simulink model "rate_limit_prove"  (R2014b)
settings: Solver=FixedStepDiscrete  StartTime=0.0  StopTime=10.0  FixedStep=0.01  RelTol=1e-3
undefined symbols (not defined in the file): sldvsubsys
libraries: sldvlib x12, simulink x6
settings Model: ModifiedByFormat=Natasha  Creator=Natasha  LastModifiedBy=Natasha
settings DebuggingCC: UnderspecifiedInitializationDetection=Classic  MergeDetectMultiDrivingBlocksExec=none
settings ConfigComp: Description=Design Verifier Custom Configuration Component  DVMode=PropertyProving  DVMaxProcessTime=1200  DVMaxTestCaseSteps=500  DVTestSuiteOptimization=CombinedObjectives (Nonlinear Extended)  DVDetectActiveLogic=on

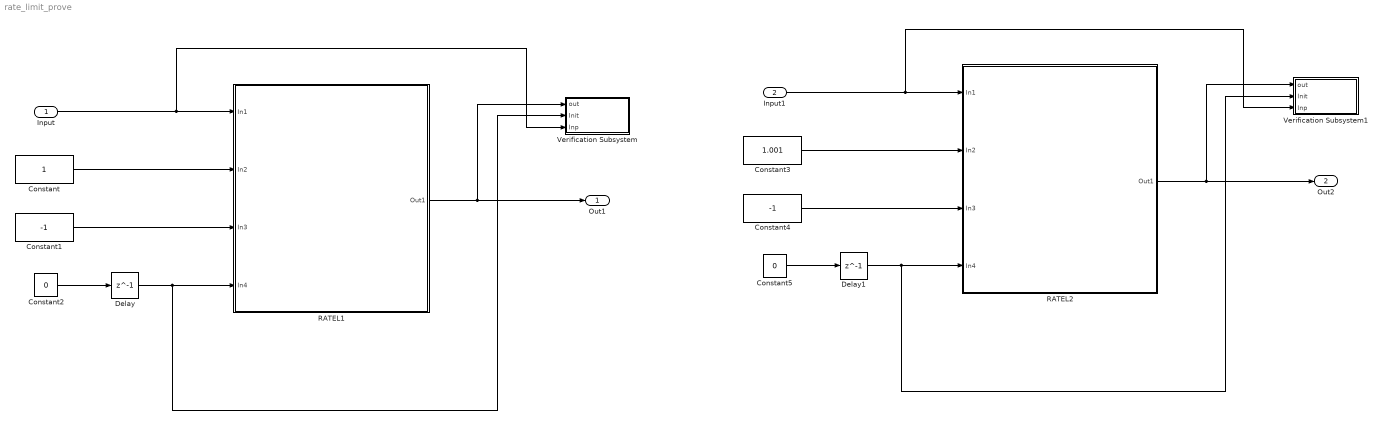
== system rate_limit_prove ==
  Input : Inport
  Input1 : Inport  Port=2
  Constant : Constant  OutDataTypeStr=single
  Constant1 : Constant  Value=-1  OutDataTypeStr=single
  Constant2 : Constant  Value=0  OutDataTypeStr=boolean
  Constant3 : Constant  Value=1.001  OutDataTypeStr=single
  Constant4 : Constant  Value=-1  OutDataTypeStr=single
  Constant5 : Constant  Value=0  OutDataTypeStr=boolean
  Delay : Delay  DelayLength=1  InitialCondition=1
  Delay1 : Delay  DelayLength=1  InitialCondition=1
  RATEL1 : Subsystem  Description=Rate Limiter  mask{DT=0.01}
      mask prompts: DT "Input the Sample Time"
      settings: AttributesFormatString=%<Description>\nSample Time = %<DT>
      mask Display:
      | port_label('output', 1, 'Rate limited')
      | port_label('input', 1, 'Input')
      | port_label('input', 2, 'Rising Limit')
      | port_label('input', 3, 'Falling Limit')
      | port_label('input', 4, 'Init')
      | patch([0.35 .5 0.65], [0 .3 0], [0 1 0])
      | text(0.4,0.1, 'Safe')
  RATEL2 : Subsystem  Description=Rate Limiter  mask{DT=0.01}
      mask prompts: DT "Input the Sample Time"
      settings: AttributesFormatString=%<Description>\nSample Time = %<DT>
      mask Display:
      | port_label('output', 1, 'Rate limited')
      | port_label('input', 1, 'Input')
      | port_label('input', 2, 'Rising Limit')
      | port_label('input', 3, 'Falling Limit')
      | port_label('input', 4, 'Init')
      | patch([0.35 .5 0.65], [0 .3 0], [0 1 0])
      | text(0.4,0.1, 'Safe')
  Verification Subsystem : Subsystem  Tag=VerificationSubsystem  DisableCoverage=on  LoadFcn=sldvsubsys('check')  TreatAsAtomicUnit=on  SimViewingDevice=on  mask(VerificationSubsystem){}
      mask init:
      | sldvsubsys('maskInit');
      settings: CopyFcn=sldvsubsys('copy');  OpenFcn=open_system(gcb,'force');
      settings: PreSaveFcn=|
      | set_param(gcb,'SimViewingDevice','on');
      | sldvsubsys('check');
      mask Help: helpview(fullfile(docroot,'toolbox','sldv','sldv.map'),'verificationsubsystem')
      mask Display: image(imread('sldvicon_versubsys.png','BackGroundColor',[1 1 1]),'center');
  Verification Subsystem1 : Subsystem  Tag=VerificationSubsystem  DisableCoverage=on  LoadFcn=sldvsubsys('check')  TreatAsAtomicUnit=on  SimViewingDevice=on  mask(VerificationSubsystem){}
      mask init:
      | sldvsubsys('maskInit');
      settings: CopyFcn=sldvsubsys('copy');  OpenFcn=open_system(gcb,'force');
      settings: PreSaveFcn=|
      | set_param(gcb,'SimViewingDevice','on');
      | sldvsubsys('check');
      mask Help: helpview(fullfile(docroot,'toolbox','sldv','sldv.map'),'verificationsubsystem')
      mask Display: image(imread('sldvicon_versubsys.png','BackGroundColor',[1 1 1]),'center');
  Out1 : Outport
  Out2 : Outport  Port=2
  wires:
  Constant/1 -> RATEL1/2(In2)
  Constant1/1 -> RATEL1/3(In3)
  Constant2/1 -> Delay/1
  RATEL1/1(Out1) -> Verification Subsystem/1(out), Out1/1
  Delay/1 -> Verification Subsystem/2(Init), RATEL1/4(In4)
  Input/1 -> RATEL1/1(In1), Verification Subsystem/3(Inp)
  Constant3/1 -> RATEL2/2(In2)
  Constant4/1 -> RATEL2/3(In3)
  Constant5/1 -> Delay1/1
  RATEL2/1(Out1) -> Verification Subsystem1/1(out), Out2/1
  Delay1/1 -> Verification Subsystem1/2(Init), RATEL2/4(In4)
  Input1/1 -> Verification Subsystem1/3(Inp), RATEL2/1(In1)

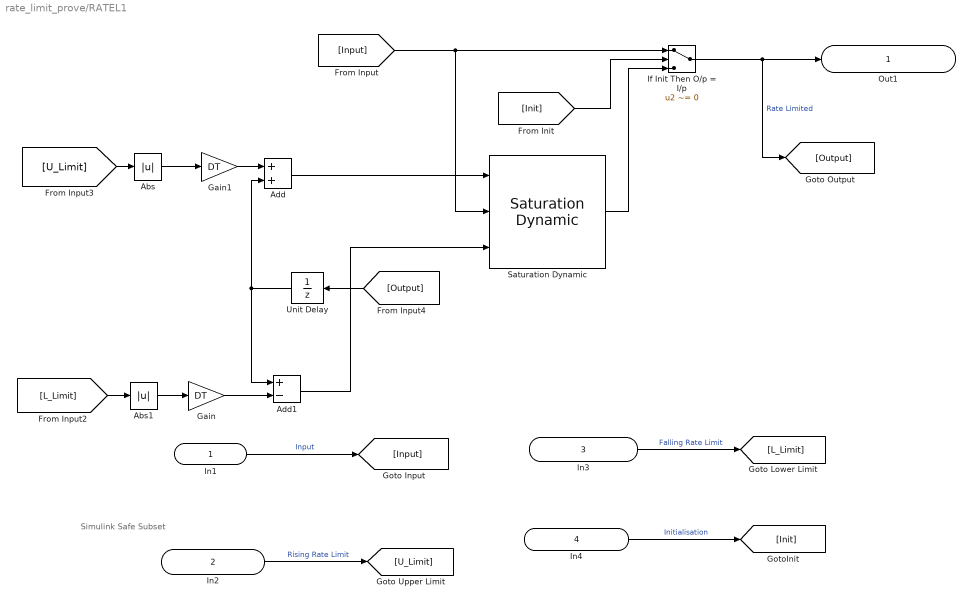
== system rate_limit_prove/RATEL1 ==
  note: Simulink
      | Safe
      | Subset
  In1 : Inport  Description=Input Signal  OutDataTypeStr=single
      settings: AttributesFormatString=%<Description>\nPort No = %<Port>\nSample Time = %<SampleTime>\nSignal Type = %<SignalType>
  In2 : Inport  Description=Rising Limit  Port=2  OutDataTypeStr=single
      settings: AttributesFormatString=%<Description>\nPort No = %<Port>\nSample Time = %<SampleTime>\nSignal Type = %<SignalType>
  In3 : Inport  Description=Falling Limit  Port=3  OutDataTypeStr=single
      settings: AttributesFormatString=%<Description>\nPort No = %<Port>\nSample Time = %<SampleTime>\nSignal Type = %<SignalType>
  In4 : Inport  Description=Initialise  Port=4  OutDataTypeStr=boolean
      settings: AttributesFormatString=%<Description>\nPort No = %<Port>\nSample Time = %<SampleTime>\nSignal Type = %<SignalType>
  Abs : Abs
      settings: AttributesFormatString=ST = %<SampleTime>
  Abs1 : Abs
      settings: AttributesFormatString=ST = %<SampleTime>
  Add : Sum
      settings: AttributesFormatString=ST = %<SampleTime>
  Add1 : Sum  Inputs=+-
      settings: AttributesFormatString=ST = %<SampleTime>
  Gain : Gain  Gain=DT
  Gain1 : Gain  Gain=DT
  If Init Then O/p = I/p : Switch  Criteria=u2 ~= 0  Threshold=0.5  ZeroCross=off
      settings: AttributesFormatString=ST = %<SampleTime>\nThreshold = %<Threshold>\n%<Criteria>
  Saturation Dynamic : simulink/Discontinuities/Saturation Dynamic  OutMin=[]  OutMax=[]  OutDataTypeStr=Inherit: Same as second input  OutDataType=fixdt(1, 16)  OutScaling=2^-10  DoSatur=off
  Unit Delay : UnitDelay  SampleTime=-1
      settings: AttributesFormatString=ST = %<SampleTime>\nInitial = %<X0>
  Out1 : Outport  Description=Output Signal
      settings: AttributesFormatString=%<Description>\nPort No = %<Port>\nSample Time = %<SampleTime>\nSignal Type = %<SignalType>
  wires:
  Add1/1 -> Saturation Dynamic/3
  Add/1 -> Saturation Dynamic/1
  [Output] -> Unit Delay/1
  Gain1/1 -> Add/1
  [U_Limit] -> Abs/1
  Unit Delay/1 -> Add1/1, Add/2
  Gain/1 -> Add1/2
  [L_Limit] -> Abs1/1
  Saturation Dynamic/1 -> If Init Then O/p = I/p/3
  If Init Then O/p = I/p/1 -> [Output], Out1/1  "Rate Limited"
  [Init] -> If Init Then O/p = I/p/2
  In4/1 -> [Init]  "Initialisation"
  In3/1 -> [L_Limit]  "Falling Rate Limit"
  In2/1 -> [U_Limit]  "Rising Rate Limit"
  In1/1 -> [Input]  "Input"
  Abs/1 -> Gain1/1
  Abs1/1 -> Gain/1
  [Input] -> If Init Then O/p = I/p/1, Saturation Dynamic/2

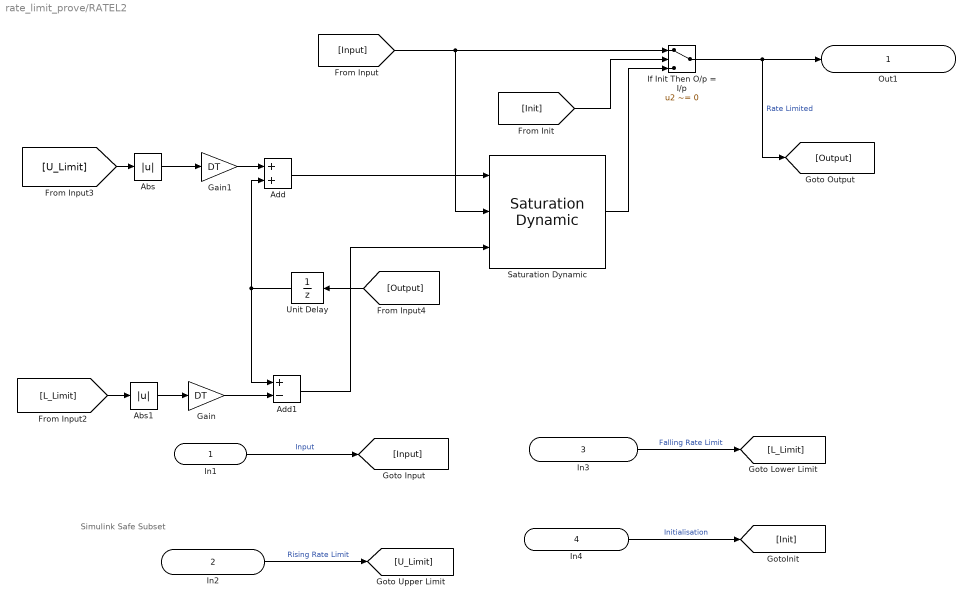
== system rate_limit_prove/RATEL2 ==
  note: Simulink
      | Safe
      | Subset
  In1 : Inport  Description=Input Signal  OutDataTypeStr=single
      settings: AttributesFormatString=%<Description>\nPort No = %<Port>\nSample Time = %<SampleTime>\nSignal Type = %<SignalType>
  In2 : Inport  Description=Rising Limit  Port=2  OutDataTypeStr=single
      settings: AttributesFormatString=%<Description>\nPort No = %<Port>\nSample Time = %<SampleTime>\nSignal Type = %<SignalType>
  In3 : Inport  Description=Falling Limit  Port=3  OutDataTypeStr=single
      settings: AttributesFormatString=%<Description>\nPort No = %<Port>\nSample Time = %<SampleTime>\nSignal Type = %<SignalType>
  In4 : Inport  Description=Initialise  Port=4  OutDataTypeStr=boolean
      settings: AttributesFormatString=%<Description>\nPort No = %<Port>\nSample Time = %<SampleTime>\nSignal Type = %<SignalType>
  Abs : Abs
      settings: AttributesFormatString=ST = %<SampleTime>
  Abs1 : Abs
      settings: AttributesFormatString=ST = %<SampleTime>
  Add : Sum
      settings: AttributesFormatString=ST = %<SampleTime>
  Add1 : Sum  Inputs=+-
      settings: AttributesFormatString=ST = %<SampleTime>
  Gain : Gain  Gain=DT
  Gain1 : Gain  Gain=DT
  If Init Then O/p = I/p : Switch  Criteria=u2 ~= 0  Threshold=0.5  ZeroCross=off
      settings: AttributesFormatString=ST = %<SampleTime>\nThreshold = %<Threshold>\n%<Criteria>
  Saturation Dynamic : simulink/Discontinuities/Saturation Dynamic  OutMin=[]  OutMax=[]  OutDataTypeStr=Inherit: Same as second input  OutDataType=fixdt(1, 16)  OutScaling=2^-10  DoSatur=off
  Unit Delay : UnitDelay  SampleTime=-1
      settings: AttributesFormatString=ST = %<SampleTime>\nInitial = %<X0>
  Out1 : Outport  Description=Output Signal
      settings: AttributesFormatString=%<Description>\nPort No = %<Port>\nSample Time = %<SampleTime>\nSignal Type = %<SignalType>
  wires:
  Add1/1 -> Saturation Dynamic/3
  Add/1 -> Saturation Dynamic/1
  [Output] -> Unit Delay/1
  Gain1/1 -> Add/1
  [U_Limit] -> Abs/1
  Unit Delay/1 -> Add1/1, Add/2
  Gain/1 -> Add1/2
  [L_Limit] -> Abs1/1
  Saturation Dynamic/1 -> If Init Then O/p = I/p/3
  If Init Then O/p = I/p/1 -> [Output], Out1/1  "Rate Limited"
  [Init] -> If Init Then O/p = I/p/2
  In4/1 -> [Init]  "Initialisation"
  In3/1 -> [L_Limit]  "Falling Rate Limit"
  In2/1 -> [U_Limit]  "Rising Rate Limit"
  In1/1 -> [Input]  "Input"
  Abs/1 -> Gain1/1
  Abs1/1 -> Gain/1
  [Input] -> If Init Then O/p = I/p/1, Saturation Dynamic/2

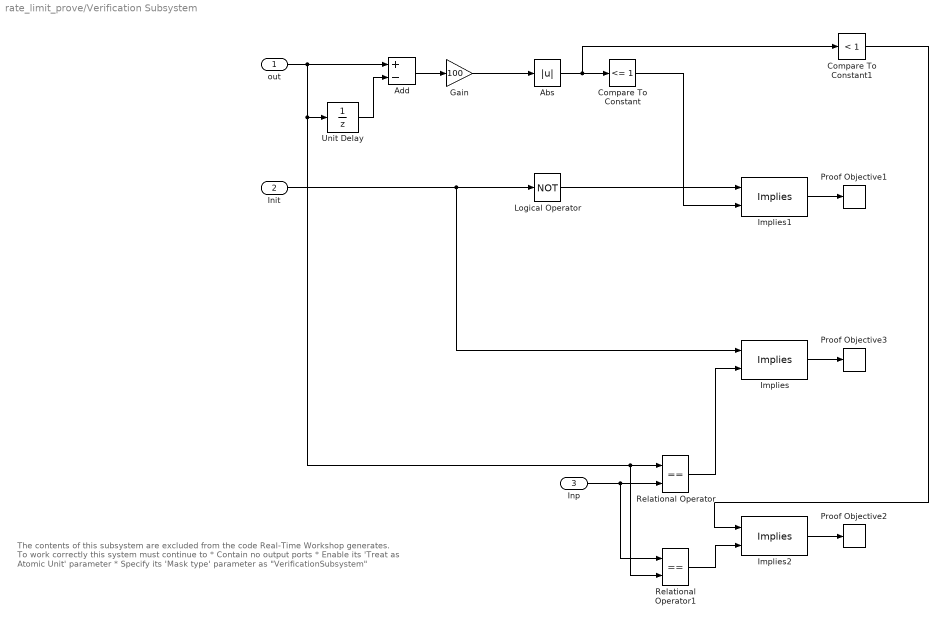
== system rate_limit_prove/Verification Subsystem ==
  note: The contents of this subsystem are excluded from the code Real-Time
      | Workshop generates.
      |
      | To work correctly this system must continue to
      | * Contain no output ports
      | * Enable its 'Treat as Atomic Unit' parameter
      | * Specify its 'Mask type' parameter as "VerificationSubsystem"
  out : Inport
  Init : Inport  Port=2
  Inp : Inport  Port=3
  Abs : Abs
  Add : Sum  Inputs=+-
  Compare To Constant : simulink/Logic and Bit Operations/Compare To Constant  relop=<=  const=1  OutDataTypeStr=boolean
  Compare To Constant1 : simulink/Logic and Bit Operations/Compare To Constant  relop=<  const=1  OutDataTypeStr=boolean
  Gain : Gain  Gain=100
  Implies : sldvlib/Verification Utilities/Implies
  Implies1 : sldvlib/Verification Utilities/Implies
  Implies2 : sldvlib/Verification Utilities/Implies
  Logical Operator : Logic  Operator=NOT  AllPortsSameDT=off  OutDataTypeStr=boolean
  Proof Objective1 : sldvlib/Objectives and Constraints/Proof Objective  enabled=on  customAVTBlockType=Proof Objective  intervals=true  dispValues=on  outEnabled=off  enableStopSim=on
      settings: AttributesFormatString=%<intervals>
  Proof Objective2 : sldvlib/Objectives and Constraints/Proof Objective  enabled=on  customAVTBlockType=Proof Objective  intervals=true  dispValues=on  outEnabled=off  enableStopSim=on
      settings: AttributesFormatString=%<intervals>
  Proof Objective3 : sldvlib/Objectives and Constraints/Proof Objective  enabled=on  customAVTBlockType=Proof Objective  intervals=true  dispValues=on  outEnabled=off  enableStopSim=on
      settings: AttributesFormatString=%<intervals>
  Relational Operator : RelationalOperator  Operator===  OutDataTypeStr=boolean
  Relational Operator1 : RelationalOperator  Operator===  OutDataTypeStr=boolean
  Unit Delay : UnitDelay  SampleTime=-1
  wires:
  Add/1 -> Gain/1
  out/1 -> Unit Delay/1, Relational Operator1/2, Relational Operator/1, Add/1
  Unit Delay/1 -> Add/2
  Gain/1 -> Abs/1
  Abs/1 -> Compare To Constant1/1, Compare To Constant/1
  Init/1 -> Implies/1, Logical Operator/1
  Relational Operator/1 -> Implies/2
  Inp/1 -> Relational Operator1/1, Relational Operator/2
  Implies/1 -> Proof Objective3/1
  Implies1/1 -> Proof Objective1/1
  Logical Operator/1 -> Implies1/1
  Compare To Constant/1 -> Implies1/2
  Implies2/1 -> Proof Objective2/1
  Relational Operator1/1 -> Implies2/2
  Compare To Constant1/1 -> Implies2/1

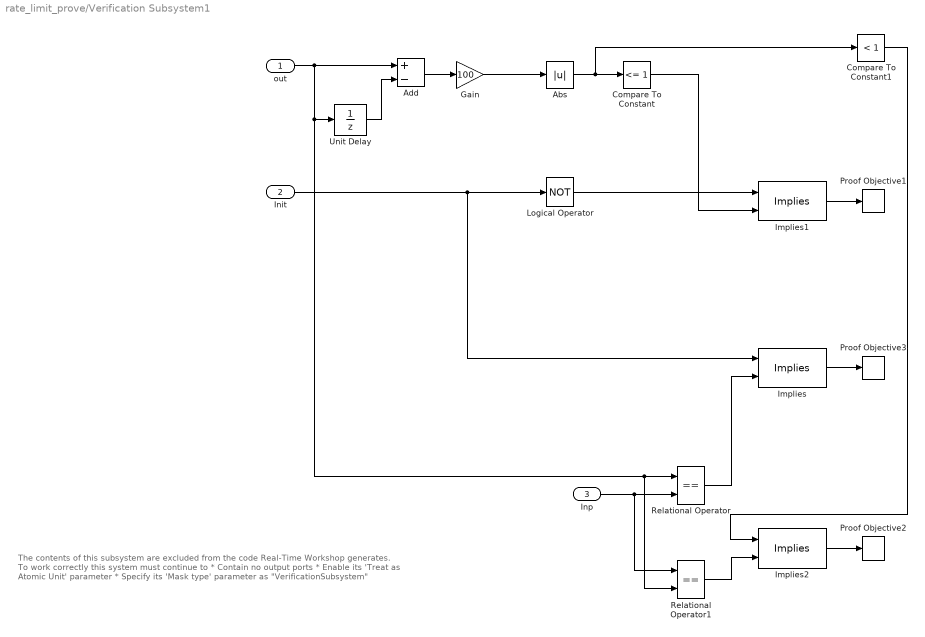
== system rate_limit_prove/Verification Subsystem1 ==
  note: The contents of this subsystem are excluded from the code Real-Time
      | Workshop generates.
      |
      | To work correctly this system must continue to
      | * Contain no output ports
      | * Enable its 'Treat as Atomic Unit' parameter
      | * Specify its 'Mask type' parameter as "VerificationSubsystem"
  out : Inport
  Init : Inport  Port=2
  Inp : Inport  Port=3
  Abs : Abs
  Add : Sum  Inputs=+-
  Compare To Constant : simulink/Logic and Bit Operations/Compare To Constant  relop=<=  const=1  OutDataTypeStr=boolean
  Compare To Constant1 : simulink/Logic and Bit Operations/Compare To Constant  relop=<  const=1  OutDataTypeStr=boolean
  Gain : Gain  Gain=100
  Implies : sldvlib/Verification Utilities/Implies
  Implies1 : sldvlib/Verification Utilities/Implies
  Implies2 : sldvlib/Verification Utilities/Implies
  Logical Operator : Logic  Operator=NOT  AllPortsSameDT=off  OutDataTypeStr=boolean
  Proof Objective1 : sldvlib/Objectives and Constraints/Proof Objective  enabled=on  customAVTBlockType=Proof Objective  intervals=true  dispValues=on  outEnabled=off  enableStopSim=on
      settings: AttributesFormatString=%<intervals>
  Proof Objective2 : sldvlib/Objectives and Constraints/Proof Objective  enabled=on  customAVTBlockType=Proof Objective  intervals=true  dispValues=on  outEnabled=off  enableStopSim=on
      settings: AttributesFormatString=%<intervals>
  Proof Objective3 : sldvlib/Objectives and Constraints/Proof Objective  enabled=on  customAVTBlockType=Proof Objective  intervals=true  dispValues=on  outEnabled=off  enableStopSim=on
      settings: AttributesFormatString=%<intervals>
  Relational Operator : RelationalOperator  Operator===  OutDataTypeStr=boolean
  Relational Operator1 : RelationalOperator  Operator===  OutDataTypeStr=boolean
  Unit Delay : UnitDelay  SampleTime=-1
  wires:
  Compare To Constant1/1 -> Implies2/1
  Relational Operator1/1 -> Implies2/2
  Implies2/1 -> Proof Objective2/1
  Compare To Constant/1 -> Implies1/2
  Logical Operator/1 -> Implies1/1
  Implies1/1 -> Proof Objective1/1
  Implies/1 -> Proof Objective3/1
  Inp/1 -> Relational Operator/2, Relational Operator1/1
  Relational Operator/1 -> Implies/2
  Init/1 -> Logical Operator/1, Implies/1
  Abs/1 -> Compare To Constant/1, Compare To Constant1/1
  Gain/1 -> Abs/1
  Unit Delay/1 -> Add/2
  out/1 -> Add/1, Relational Operator/1, Relational Operator1/2, Unit Delay/1
  Add/1 -> Gain/1
